simulink library "libsb2sl"  (Simulink 7.3)
settings: Solver=ode45  SolverMode=SingleTasking  StartTime=0.0  StopTime=10.0  RelTol=1e-3
PostLoadFcn:
  | setsysloc libsb2sl
undefined symbols (not defined in the file): A, Ac, Ad, B, Bc, Bd, C, Cc, Cd, code, const, D, data, Dc, Dd, DiscIntNeverNeededParam, gain, info, k, m, map, no, stat, X0, xd, xi
libraries: simulink3 x17, simulink x5, libsb2sl x3
(part 1 of 3)
Description:
  | Translation blocks
  | 
  | Copyright 1997-2008 The MathWorks, Inc.
settings Model: Creator=alex  LastModifiedBy=sgage  ExtModeAutoUpdateStatusClock=off
settings Model: ForwardingTableString=|
  | ||__slOldName__||libsb2sl/TRN/Sph2Cart||__slNewName__||simulink_extras/Transformations/Spherical to
  | Cartesian||__slOldName__||libsb2sl/TRN/Cart2Sph||__slNewName__||simulink_extras/Transformations/Cartesian to
  | Spherical||__slOldName__||libsb2sl/TRN/Polar2Cart||__slNewName__||simulink_extras/Transformations/Polar to
  | Cartesian||__slOldName__||libsb2sl/TRN/Cart2Polar||__slNewName__||simulink_extras/Transformations/Cartesian to
  | Polar||__slOldName__||libsb2sl/ALG/DotProduct||__slNewName__||simulink/Math
  | Operations/Dot Product

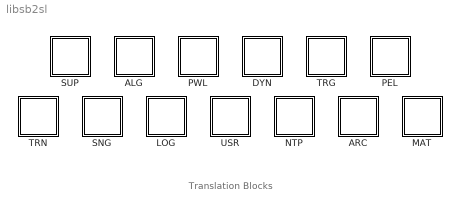
== system libsb2sl ==
  note: Translation Blocks
  ALG : Subsystem
  ARC : Subsystem
  DYN : Subsystem
  LOG : Subsystem
  MAT : Subsystem  AncestorBlock=libsb2sl/ARC
  NTP : Subsystem
  PEL : Subsystem
  PWL : Subsystem
  SNG : Subsystem
  SUP : Subsystem
  TRG : Subsystem
  TRN : Subsystem
  USR : Subsystem

== system libsb2sl/ALG ==
  1VarPoly : S-Function  FunctionName=sb1varpoly  Parameters=COEFF  EnableBusSupport=off  mask(ALG-Palette){COEFF=[1 2]}
      mask prompts: COEFF "Coefficients:"
      mask init:
      | [x,y]=sblibico('polyOneVar');
      mask Display: plot(0,0,1,1,x,y)
  AlgExpression : Subsystem
  CrossProd : Subsystem  mask(ALG-Palette){}
      mask help: Cross-product multiplication.
      mask init:
      | [x,y]=sblibico('crossProduct');
      mask Display: plot(0,0,1,1,x,y)

== system libsb2sl/ARC ==
  BreakPoints : Subsystem  mask(ARC-Palette){BrkPoints=[-1 1;0 2;1 3]}
      mask prompts: BrkPoints "Breakpoint Matrix:"
      mask help: Linear Interpolation.
      mask init:
      | % LinInterp MaskInit code
      | [x,y]=sblibico('linearInterp');
      | in1BrkPoints=BrkPoints(:,1:2:end);
      | outBrkPoints=BrkPoints(:,2:2:end);
      mask Display: plot(0,0,1,1,x,y)
  InterpTable : Subsystem  mask(ARC-Palette){numInp=One, BrkPoints=[-5:5; -5:5; -10:2:10]'}
      mask prompts: numInp "Number of Inputs:"; BrkPoints "Interpolation Table:"
      mask help: Linear Interpolation Table.
      mask init:
      | if (numInp==1)
      | in1BrkPoints=BrkPoints(:,1);
      | in2BrkPoints=[1:size(BrkPoints,2)-1];
      | outBrkPoints=BrkPoints(:,2:end);
      | [x,y]=sblibico('linearInterp');
      | else
      | in1BrkPoints=BrkPoints(1:end-1,1);
      | in2BrkPoints=BrkPoints(end,2:end);
      | outBrkPoints=BrkPoints(1:end-1,2:end);
      | [x,y]=sblibico('bilinearInterp');
      | end
      mask StyleString: popup(One|Two),edit
      mask Display: plot(0,0,1,1,x,y)

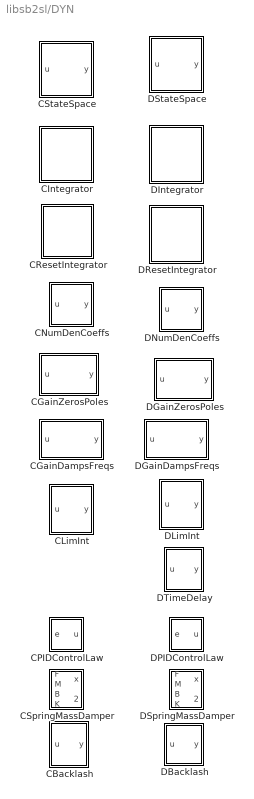
== system libsb2sl/DYN ==
  CBacklash : Subsystem  mask(DYN-Palette){W=1, N=1, X0=0, Wc=1}
      mask prompts: W "Backlash Width:"; N "Backlash Slope:"; X0 "Initial Conditions:"; Wc "Cutoff Frequency:"
      mask help: A non-linear dynamic system that models hysteresis.
      mask init:
      | lb=-0.5*W; ub=-lb;
      | [x,y]=sblibico('backlash');
      mask Display: plot(0,0,1,1,x,y)
  CGainDampsFreqs : Subsystem  mask(DYN-Palette){G=1, Xz=[], Wz=[], Xp=[0.7], Wp=[1], Y0=0}
      mask prompts: G "Gain:"; Xz "Zeros-Damping Ratios:"; Wz "Zeros-Natural Frequencies:"; Xp "Poles-Damping Ratios:"; Wp "Poles-Natural Frequencies:"; Y0 "Initial Output:"
      mask help: Transfer function in damping ratios and natural frequencies.
      mask init:
      | [A,B,C,D]=sblibdrv('CmplxZP',G,Xz,Wz,Xp,Wp,0);
      | if (isempty(Y0)), Y0 = zeros(1,size(C,1)); end;
      | X0=C\Y0;
      | [x,y]=sblibico('gainDampsFreq','cont');
      mask Display: plot(0,0,1,1,x,y)
  CGainZerosPoles : Subsystem  mask(DYN-Palette){K=1, Z=1, P=-1, Y0=0}
      mask prompts: K "Gain:"; Z "Zeros:"; P "Poles:"; Y0 "Initial Output:"
      mask help: Transfer function expressed in real poles and real zeros.
      mask init:
      | [A,B,C,D]=zp2ss(Z,P,K);
      | if (isempty(Y0)), X0 = zeros(1,size(C,1)); end;
      | X0=C\Y0;
      | [x,y]=sblibico('gainZerosPoles','cont');
      mask Display: plot(0,0,1,1,x,y)
  CIntegrator : Subsystem
  CLimInt : Subsystem  mask(DYN-Palette){UB=5, LB=-5, K=1, X0=5}
      mask prompts: UB "Upper Limit:"; LB "Lower Limit:"; K "Gain:"; X0 "Initial condition:"
      mask init:
      | [x,y]=sblibico('limIntegrator','cont');
      mask Display: plot(0,0,1,1,x,y)
  CNumDenCoeffs : Subsystem  mask(DYN-Palette){NU=2, NUM=[1 2;1.1 1], DEN=[0.5  1], Y0=[0.5;0.5]}
      mask prompts: NU "Number of Inputs:"; NUM "Numerator:"; DEN "Denominator:"; Y0 "Initial Output:"
      mask help: Transfer function in numerator-denominator form.
      mask init:
      | if (isempty(NU)), NU=1; end
      | [Ac,Bc,Cc,Dc] = sblibdrv('NumDen',NUM,DEN,NU);
      | if (isempty(Y0)); Y0=zeros(1,size(Cc,1)); end
      | X0=Cc\Y0(:);
      | [x,y]=sblibico('numDenCoeffs','cont');
      mask Display: plot(0,0,1,1,x,y)
  CPIDControlLaw : Subsystem  mask(DYN-Palette){P=1, I=1, D=0, TAU=0, X0=0}
      mask prompts: P "Proportional Gain:"; I "Integral Gain:"; D "Derivative Gain:"; TAU "Derivative Time Constant:"; X0 "Initial Conditions:"
      mask help: PID Control Law.
      mask init:
      | if (exist('X0')==0),X0=[];end
      | [xi,xd]=sblibdrv('pidControl',I,D,TAU,X0);
      | [x,y]=sblibico('pidControl');
      mask Display: plot(0,0,1,1,x,y)
  CResetIntegrator : Subsystem
  CSpringMassDamper : Subsystem  mask(DYN-Palette){X0=[0,0]}
      mask prompts: X0 "Initial Conditions:"
      mask help: Spring Mass Damper.
      mask init:
      | [x,y]=sblibico('springMassDamper');
      mask Display: plot(0,0,1,1,x,y)
  CStateSpace : Subsystem  mask(DYN-Palette){NX=1, SYS=[1 1;1 0], X0=[]}
      mask prompts: NX "Number of States:"; SYS "System Matrix:"; X0 "Initial Conditions:"
      mask help: State-space system.
      mask init:
      | if (~exist('X0','var')), X0=[]; end
      | if isempty(X0), X0=zeros(NX,1); end
      | NX1=NX+1;
      | A=SYS(1:NX,1:NX);
      | B=SYS(1:NX,NX1:end);
      | C=SYS(NX1:end,1:NX);
      | D=SYS(NX1:end,NX1:end);
      | [x,y]=sblibico('stateSpace','cont');
      mask Display: plot(0,0,1,1,x,y)
  DBacklash : Subsystem  mask(DYN-Palette){W=1, N=1, X0=0, TS=1}
      mask prompts: W "Backlash Width:"; N "Backlash Slope:"; X0 "Initial Conditions:"; TS "Sampling Time:"
      mask help: A non-linear dynamic system that models hysteresis.
      mask init:
      | lb=-0.5*W; ub=-lb;
      | [x,y]=sblibico('backlash');
      mask Display: plot(0,0,1,1,x,y)
  DGainDampsFreqs : Subsystem  mask(DYN-Palette){G=1, Xz=[], Wz=[], Xp=0.7, Wp=1, Y0=0, TS=0.1}
      mask prompts: G "Gain:"; Xz "Zeros-Damping Ratios:"; Wz "Zeros-Natural Frequencies:"; Xp "Poles-Damping Ratios:"; Wp "Poles-Natural Frequencies:"; Y0 "Initial Output:"; TS "Sample Time:"
      mask help: Transfer function in damping ratios and natural frequencies.
      mask init:
      | [A,B,C,D]=sblibdrv('CmplxZP',G,Xz,Wz,Xp,Wp,TS(1));
      | if (isempty(Y0)), Y0 = zeros(1,size(C,1)); end;
      | X0=C\Y0;
      | [x,y]=sblibico('gainDampsFreq','disc');
      mask Display: plot(0,0,1,1,x,y)
  DGainZerosPoles : Subsystem  mask(DYN-Palette){K=1, Z=[], P=-1, Y0=0, TS=1}
      mask prompts: K "Gain:"; Z "Zeros:"; P "Poles:"; Y0 "Initial Output:"; TS "Sample Time:"
      mask help: Transfer function expressed in real poles and real zeros.
      mask init:
      | [A,B,C,D]=zp2ss(Z,P,K);
      | if (isempty(Y0)), Y0 = zeros(1,size(C,1)); end;
      | X0=C\Y0;
      | [x,y]=sblibico('gainZerosPoles','disc');
      mask Display: plot(0,0,1,1,x,y)
  DIntegrator : Subsystem
  DLimInt : Subsystem  mask(DYN-Palette){IMODE=ForwardEuler, UB=5, LB=-5, K=1, X0=0, TS=0.1}
      mask prompts: IMODE "Integrator Method:"; UB "Upper Limit:"; LB "Lower Limit:"; K "Gain:"; X0 "Initial Conditions:"; TS "Sampling Period:"
      mask init:
      | method={'ForwardEuler';'BackwardEuler';'Trapezoidal'};
      | set_param([gcb '/Integrator'],'IntegratorMethod',method{IMODE});
      | [x,y]=sblibico('limIntegrator','disc');
      mask StyleString: popup(ForwardEuler|BackwardEuler|Trapezoidal),edit,edit,edit,edit,edit
      mask Display: plot(0,0,1,1,x,y)
  DNumDenCoeffs : Subsystem  mask(DYN-Palette){NU=2, NUM=[1 2;1.1 1], DEN=[0.5  1], Y0=-[0.5;0.5], TS=0.1}
      mask prompts: NU "Number of Inputs:"; NUM "Numerator:"; DEN "Denominator:"; Y0 "Initial Output:"; TS "Sample Time:"
      mask help: Transfer function in numerator-denominator form.
      mask init:
      | if (isempty(NU)), NU=1; end
      | [Ad,Bd,Cd,Dd]=sblibdrv('NumDen',NUM,DEN,NU);
      | if (isempty(Y0)); Y0=zeros(1,size(Cd,1)); end
      | X0=Cd\Y0(:);
      | [x,y]=sblibico('numDenCoeffs','disc');
      mask Display: plot(0,0,1,1,x,y)
  DPIDControlLaw : Subsystem  mask(DYN-Palette){P=1, I=1, D=0, TAU=0, X0=0, TS=1}
      mask prompts: P "Proportional Gain:"; I "Integral Gain:"; D "Derivative Gain:"; TAU "Derivative Time Constant:"; X0 "Initial Conditions:"; TS "Sampling Period:"
      mask help: PID Control Law.
      mask init:
      | if (exist('X0')==0),X0=[];end
      | [xi,xd]=sblibdrv('pidControl',I,D,TAU,X0);
      | [x,y]=sblibico('pidControl');
      mask Display: plot(0,0,1,1,x,y)
  DResetIntegrator : Subsystem
  DSpringMassDamper : Subsystem  mask(DYN-Palette){X0=[0,0], TS=0.01}
      mask prompts: X0 "Initial Conditions:"; TS "Sampling Period:"
      mask help: Spring Mass Damper.
      mask init:
      | if (length(TS)==1),TS(2)=0;end
      | [x,y]=sblibico('springMassDamper');
      mask Display: plot(0,0,1,1,x,y)
  DStateSpace : Subsystem  mask(DYN-Palette){NX=1, SYS=[1 1;1 0], X0=[], TS=1}
      mask prompts: NX "Number of States:"; SYS "System Matrix:"; X0 "Initial Conditions:"; TS "Sampling Time:"
      mask init:
      | if (~exist('X0','var')), X0=[]; end
      | if isempty(X0), X0=zeros(NX,1); end
      | NX1=NX+1;
      | A=SYS(1:NX,1:NX);
      | B=SYS(1:NX,NX1:end);
      | C=SYS(NX1:end,1:NX);
      | D=SYS(NX1:end,NX1:end);
      | [x,y]=sblibico('stateSpace','disc');
      mask Display: plot(0,0,1,1,x,y)
  DTimeDelay : Subsystem  mask(DYN-Palette){TAU=1.1, Y0=0, TS=1}
      mask prompts: TAU "Time Delay:"; Y0 "Initial Output:"; TS "Sampling Time:"
      mask init:
      | if (isempty(Y0)), Y0=0; end;
      | [k,m,no,X0]=sblibdrv('dDelay',TAU,Y0,TS);
      | [x,y]=sblibico('timeDelay');
      mask Display: plot(0,0,1,1,x,y)

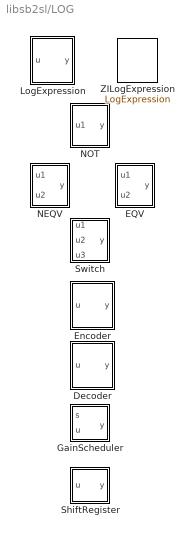
== system libsb2sl/LOG ==
  Decoder : Subsystem  mask(LOG-Palette){BPI=4, MIN=-1, MAX=1}
      mask prompts: BPI "Number of Bits per Input:"; MIN "Input Minimum:"; MAX "Input Maximum:"
      mask help: Decimal to binary conversion.
      mask init:
      | [x,y]=sblibico('decoder');
      mask Display: plot(0,0,1,1,x,y)
  EQV : Subsystem  mask(LOG-Palette){}
      mask help: Logical operator EQV.
      mask init:
      | [x,y]=sblibico('logOperator','EQV');
      mask Display: plot(0,0,1,1,x,y)
  Encoder : Subsystem  mask(LOG-Palette){BPO=4, MIN=-1, MAX=1}
      mask prompts: BPO "Number of Bits per Output:"; MIN "Output Minimum:"; MAX "Output Maximum:"
      mask help: Binary to decimal conversion.
      mask init:
      | [x,y]=sblibico('encoder');
      mask Display: plot(0,0,1,1,x,y)
  GainScheduler : Subsystem  mask(LOG-Palette){IND=[-1,0,1], GAIN=[1,2,3]}
      mask prompts: IND "Switch Breakpoints:"; GAIN "Gain Matrices:"
      mask help: Gain scheduler
      mask init:
      | [x,y]=sblibico('gainSched');
      mask Display: plot(0,0,1,1,x,y)
  LogExpression : Subsystem  mask(LOG-Palette){SRC='y1=u1;y2=t;', P0=[], TS=-1}
      mask prompts: SRC "Logical and Relational Equations:"; P0 "Initial Parameter Values:"; TS "Sampling Period:"
      mask help: Logical expressions.
      mask init:
      | if (exist('P0')==0),P0=[];end
      | [src,stat,code,data,info]=sblibdrv('LogicalExp',SRC,P0);
      mask Display: text(0.1,0.5,src,'HorizontalAlignment','left')
  NEQV : Subsystem  mask(LOG-Palette){}
      mask help: Logical operator NEQV.
      mask init:
      | [x,y]=sblibico('logOperator','NEQV');
      mask Display: plot(0,0,1,1,x,y)
  NOT : Subsystem  mask(LOG-Palette){}
      mask help: Logical operator NOT.
      mask init:
      | [x,y]=sblibico('logOperator','NOT');
      mask Display: plot(0,0,1,1,x,y)
  ShiftRegister : Subsystem  mask(LOG-Palette){NX=1, NY=1, X0=0, TS=1}
      mask prompts: NX "Number of Stages:"; NY "Number of  Output Stages:"; X0 "Initial Values:"; TS "Sampling Time:"
      mask help: Sequential Shift Register
      mask init:
      | if (~exist('X0','var')), X0=[]; end
      | if (isempty(X0)), X0=zeros(NX,1); end
      | [x,y]=sblibico('shiftReg');
      mask Display: plot(0,0,1,1,x,y)
  Switch : Subsystem
      mask Type: LOG-Palette
      mask Description: Switches between two data sources.
      mask Display: plot(0,1.2,10,10.5,[0 5 5 4.5 5.5 5],[9 9 4 5.5 5.5 4],[0 3],[6 6],[0 3 8 10],[3 3 6 6])
  ZILogExpression : libsb2sl/LOG/LogExpression  SystemSampleTime=-1  SRC='y1=u1;y2=t;'  P0=[]  TS=-1

== system libsb2sl/MAT ==
  Constant : Subsystem  mask(MAT-Palette){constantName='H', constantValue=[1,1;2,4];}
      mask prompts: constantName "Constant Name:"; constantValue "Constant Value:"
      mask init:
      | if (~exist('constantName','var')), constantName='';end
      | if (isempty(constantName)), constantName='H';end
      | if (~ischar(constantName)), constantName=char(constantName);end
      | if (any(size(constantValue) > 1)), constantValue=constantValue.';constantValue=constantValue(:);end
      mask Display: disp(constantName)
  LeftMultiply : Subsystem  mask(MAT-Palette){G=[5 10], dimMatrixA=[2,2]}
      mask prompts: G "Gain:"; dimMatrixA "Matrix A Dimension:"
      mask init:
      | [x,y]=sblibico('matLeftMul');
      | nARows=dimMatrixA(1);nACols=dimMatrixA(2);
      | [nGRows,nGCols]=size(G);
      | G=G.';
      | if (nGCols ~= nARows)
      | error('Inner matrix dimensions must agree.');
      | end
      mask Display: plot(0,0,1,1,x,y)
  MatLeftDivide : Subsystem  mask(MAT-Palette){dimMatrixA=[2,2], dimMatrixB=[2,2]}
      mask prompts: dimMatrixA "Matrix A Dimension:"; dimMatrixB "Matrix B Dimension:"
      mask init:
      | [x,y]=sblibico('matLeftDiv');
      | nARows=dimMatrixA(1);nACols=dimMatrixA(2);
      | nBRows=dimMatrixB(1);nBCols=dimMatrixB(2);
      | if (nACols ~= nBRows)
      | error('Matrix dimensions must agree.');
      | end
      mask Display: plot(0,0,1,1,x,y)
  MatRightDivide : Subsystem  mask(MAT-Palette){dimMatrixA=[2,2], dimMatrixB=[2,2]}
      mask prompts: dimMatrixA "Matrix A Dimension:"; dimMatrixB "Matrix B Dimension:"
      mask init:
      | [x,y]=sblibico('matRightDiv');
      | nARows=dimMatrixA(1);nACols=dimMatrixA(2);
      | nBRows=dimMatrixB(1);nBCols=dimMatrixB(2);
      | if (nARows ~= nBCols)
      | error('Matrix dimensions must agree.');
      | end
      mask Display: plot(0,0,1,1,x,y)
  MatrixInverse : Subsystem  mask(MAT-Palette){dimMatrixA=[2,2]}
      mask prompts: dimMatrixA "Matrix A Dimension:"
      mask init:
      | [x,y]=sblibico('matInverse');
      | nARows=dimMatrixA(1);nACols=dimMatrixA(2);
      mask Display: plot(0,0,1,1,x,y)
  MatrixMultiply : Subsystem  mask(MAT-Palette){dimMatrixA=[2,2], dimMatrixB=[2,2]}
      mask prompts: dimMatrixA "Matrix A Dimension:"; dimMatrixB "Matrix B Dimension:"
      mask init:
      | [x,y]=sblibico('matMultiply');
      | nARows=dimMatrixA(1);nACols=dimMatrixA(2);
      | nBRows=dimMatrixB(1);nBCols=dimMatrixB(2);
      | if (nACols ~= nBRows)
      | error('Inner matrix dimensions must agree.');
      | end
      mask Display: plot(0,0,1,1,x,y)
  MatrixTranspose : Subsystem  mask(MAT-Palette){dimMatrixA=[2,2]}
      mask prompts: dimMatrixA "Matrix A Dimension:"
      mask init:
      | [x,y]=sblibico('matTrans');
      | nARows=dimMatrixA(1);nACols=dimMatrixA(2);
      | if ((nARows==1)|(nACols==1)),
      | mapIndices=1:nARows*nACols;
      | else
      | mapMatrix=[1:nACols;nACols*ones(nARows-1,nACols)];
      | mapIndices=cumsum(mapMatrix);
      | end
      mask Display: plot(0,0,1,1,x,y)
  RightMultiply : Subsystem  mask(MAT-Palette){dimMatrixA=[2,2], G=[5; 10]}
      mask prompts: dimMatrixA "Matrix A Dimension:"; G "Gain:"
      mask init:
      | [x,y]=sblibico('matRightMul');
      | nARows=dimMatrixA(1);nACols=dimMatrixA(2);
      | [nGRows,nGCols]=size(G);
      | G=G.';
      | if (nACols ~= nGRows)
      | error('Inner matrix dimensions must agree.');
      | end
      mask Display: plot(0,0,1,1,x,y)

== system libsb2sl/NTP ==
  BiCubicInterp : Subsystem  mask(NTP-Palette){in1BrkPoints=[-1,1], in2BrkPoints=[-1,0,1], outBrkPoints=[-1,1;-1,1;-1,1]}
      mask prompts: in1BrkPoints "Input-1 Breakpoints:"; in2BrkPoints "Input-2 Breakpoints:"; outBrkPoints "Output Values:"
      mask help: Bicubic interpolation.
      mask init:
      | % BiCubicInterp MaskInit code
      | [x,y]=sblibico('bicubicInterp');
      mask Display: plot(0,0,1,1,x,y)
  BiLinearInterp : Subsystem  mask(NTP-Palette){in1BrkPoints=[-1,1], in2BrkPoints=[-1,0,1], outBrkPoints=[-1,1;-1,1;-1,1]}
      mask prompts: in1BrkPoints "Input-1 Breakpoints:"; in2BrkPoints "Input-2 Breakpoints:"; outBrkPoints "Output Values:"
      mask help: Bilinear interpolation.
      mask init:
      | % BiLinInterp MaskInit code
      | [x,y]=sblibico('bilinearInterp');
      | 
      | % Set up for sfun_lookupnd input
      | bpData = [in2BrkPoints(:); in1BrkPoints(:)];  % Note: row major!
      | bpIndices_uint32 = uint32([0, length(in2BrkPoints)]);
      | searchMode = 2;
      | cacheBpFlag = 1;
      | tableData = outBrkPoints;
      | numDims = 2;
      | interpMethod = 2;
      | extrapMethod = 2;
      | rangeErrorMode = 1;
      | vectorInputFlag = 0;
      mask Display: plot(0,0,1,1,x,y)
  ConstantInterp : Subsystem  mask(NTP-Palette){in1BrkPoints=[-1,0,1], outBrkPoints=[1,2,3]}
      mask prompts: in1BrkPoints "Input Breakpoints:"; outBrkPoints "Output Values:"
      mask help: Constant Interpolation.
      mask init:
      | % ConstantInterp MaskInit code
      | [x,y]=sblibico('constInterp');
      mask Display: plot(0,0,1,1,x,y)
  CubicInterp : Subsystem  mask(TRN-Palette){in1BrkPoints=[-1,0,1], outBrkPoints=[1,2,3]}
      mask prompts: in1BrkPoints "Input Breakpoints:"; outBrkPoints "Output Values:"
      mask help: Cubic Spline Interpolation
      mask init:
      | %CubicInterp MaskInit code
      | [x,y]=sblibico('cubicInterp');
      mask Display: plot(0,0,1,1,x,y)
  LinearInterp : Subsystem  mask(TRN-Palette){in1BrkPoints=[-1,0,1], outBrkPoints=[1,2,3]}
      mask prompts: in1BrkPoints "Input Breakpoints:"; outBrkPoints "Output Values:"
      mask help: Linear Interpolation.
      mask init:
      | % LinInterp MaskInit code
      | [x,y]=sblibico('linearInterp');
      mask Display: plot(0,0,1,1,x,y)
  MultiLinearInterp : Subsystem  mask(NTP-Palette){NINP=2, in1BrkPoints=[1,2], in2BrkPoints=[1,2], in3BrkPoints=3, in4BrkPoints=4, in5BrkPoints=5, in6BrkPoints=6, in7BrkPoints=7, in8BrkPoints=8, outBrkPoints=[1,2;3,4]}
      mask prompts: NINP "Number of  Inputs:"; in1BrkPoints "Input-1 Breakpoints:"; in2BrkPoints "Input-2 Breakpoints:"; in3BrkPoints "Input-3 Breakpoints:"; in4BrkPoints "Input-4 Breakpoints:"; in5BrkPoints "Input-5 Breakpoints:"; in6BrkPoints "Input-6 Breakpoints:"; in7BrkPoints "Input-7 Breakpoints:"; in8BrkPoints "Input-8 Breakpoints:"; outBrkPoints "Output Values:"
      mask help: Multilinear interpolation.
      mask init:
      | % MultiLinInterp MaskInit code
      | [x,y]=sblibico('mdlinearInterp',NINP);
      | 
      | % Set up for sfun_lookupnd input
      | bpSizes = zeros(1,NINP+1);
      | bpSizes(1) = length(in1BrkPoints);
      | for i = 1:NINP,  % NINP is 1 for 2D, 2 for 3D, etc.
      |   bpDataNext = eval(['in' num2str(i+1) 'BrkPoints(:)']);
      |   bpSizes(i+1) = length(bpDataNext);
      |  end
      | tableData = reshape(outBrkPoints,bpSizes);
      mask StyleString: popup(2|3|4|5|6|7|8),edit,edit,edit,edit,edit,edit,edit,edit,edit
      mask CallbackString: sblibdrv('MultiLin','mask',gcb);|||||||||
      mask Display: plot(0,0,1,1,x,y)

== system libsb2sl/PEL ==
  Constant**u : Subsystem  mask(PEL-Palette){CONST=5}
      mask prompts: CONST "Constant:"
      mask init:
      | [x,y]=sblibico('constantU');
      mask Display: plot(0,0,1,1,x,y)
  SignedSqrt : Subsystem  mask(PEL-Palette){}
      mask init:
      | [x,y]=sblibico('signedSqrt');
      mask Display: plot(0,0,1,1,x,y)
  u**Constant : Subsystem  mask(PEL-Palette){CONST=5}
      mask prompts: CONST "Constant:"
      mask init:
      | [x,y]=sblibico('uConstant');
      mask Display: plot(0,0,1,1,x,y)

== system libsb2sl/PWL ==
  Preload : Subsystem  mask(PWL-Palette){preload=[1 3 2 0], slope=1}
      mask help: Performs preload or Coulomb switch function.
      mask init:
      | x=max(preload(1),slope(1)+preload(1));
      mask Display: plot([-1 0 0 1],[-slope(1)-preload(1),-preload(1),preload(1), slope(1)+preload(1)],[-1 1],[0 0],[0 0],[-x,x])
  Quantization : Subsystem  mask(PWL-Palette){RES=1, OPER=round}
      mask prompts: RES "Resolution:"; OPER "Type"
      mask init:
      | x=[-3:0.1:3];operator={'round';'fix';'floor';'ceil'};
      | y=feval(operator{OPER},x);
      | [xx,yy]=stairs(x,y);
      | set_param([gcb '/Type'],'Operator',operator{OPER});
      mask StyleString: edit,popup(round|truncate|floor|ceil)
      mask Display: plot([0 0],[-3,3],[-3,3],[0 0],xx,yy)

== system libsb2sl/SNG ==
  CNormalRandom : Subsystem  mask(SGN-Palette){SEED=0, T0=0, MEAN=0, STD=1, INTM=Linear, TS=1}
      mask prompts: T0 "Relative Start Time:"; STD "Standard Deviation:"; INTM "Interpolation Method:"; TS "Output Interval:"
      mask help: Random Number Generator, Normal
      mask init:
      | start=sscanf(get_param(bdroot(gcs),'StartTime'),'%g')+T0;
      mask StyleString: edit,edit,edit,edit,popup(Constant|Linear),edit
      mask Display: plot([-1,11],[0,0],[0,0],[-0.1,1],[0:10],rand(1,11))
  CUniformRandom : Subsystem  mask(SGN-Palette){SEED=1, T0=0, MIN=0, MAX=1, INTM=Constant, TS=1}
      mask prompts: T0 "Relative Start Time:"; MIN "Minimum:"; MAX "Maximum:"; INTM "Interpolation Method:"; TS "Output Interval:"
      mask help: Random Number Generator, Uniform.
      mask init:
      | start=sscanf(get_param(bdroot(gcs),'StartTime'),'%g')+T0;
      mask StyleString: edit,edit,edit,edit,popup(Constant|Linear),edit
      mask Display: plot([-1,11],[0,0],[0,0],[-0.1,1],[0:10],rand(1,11))
  DNormalRandom : Subsystem  mask(SGN-Palette){SEED=0, T0=0, MEAN=0, STD=1, TS=1}
      mask prompts: T0 "Relative Start Time:"; STD "Standard Deviation:"; TS "Sampling Time:"
      mask help: Random Number Generator, Normal
      mask init:
      | start=sscanf(get_param(bdroot(gcs),'StartTime'),'%g')+T0;
      mask Display: plot([-1,11],[0,0],[0,0],[-0.1,1],[0:10],rand(1,11))
  DUniformRandom : Subsystem  mask(SGN-Palette){SEED=1, T0=0, MIN=0, MAX=1, TS=1}
      mask prompts: T0 "Relative Start Time:"; MIN "Minimum:"; MAX "Maximum:"; TS "Sampling Time:"
      mask help: Random Number Generator, Uniform.
      mask init:
      | start=sscanf(get_param(bdroot(gcs),'StartTime'),'%g')+T0;
      mask Display: plot([-1,11],[0,0],[0,0],[-0.1,1],[0:10],rand(1,11))
  GenWaveform : Subsystem  mask(SGN-Palette){T0=0.6, TAC=[0 1 2], SAC=[0 0;1 2;0 0]}
      mask prompts: T0 "Relative Start Time:"; TAC "Time Values:"; SAC "Output Values:"
      mask help: General Waveform.
      mask init:
      | in1BrkPoints=TAC(:);
      | outBrkPoints=SAC;
      | period = max(in1BrkPoints);
      | start=sscanf(get_param(bdroot(gcs),'StartTime'),'%g')+T0;
      mask Display: plot([1,1,1,11],[-1,2,0,0],[3,4,4.5,5,6,7,8,8.5,9,10,11],[0,1,0.8,1.5,-0.5,0,1,0.8,1.5,-0.5,0])
  LimRamp : Subsystem  mask(SGN-Palette){T0=[2 4], RATE=[1 -1], LMT=no, SAT=[]}
      mask prompts: T0 "Relative Start Time:"; RATE "Ramp Signal Slope:"; LMT "Should Ramp be Limited?"; SAT "Ramp Saturation:"
      mask help: Ramp (Limited)
      mask init:
      | if (LMT==1),SAT=RATE*(sscanf(get_param(bdroot(gcs),'StopTime'),'%g')+1);end;
      | start=sscanf(get_param(bdroot(gcs),'StartTime'),'%g')+T0;
      mask StyleString: edit,edit,popup(no|yes),edit
      mask Display: plot([1,1,1,10],[-1,6,0,0],[3,9,10],[0,5,5])
  PulseTrain : Subsystem  mask(SNG-Palette){T0=[2 3], A=[1 0.8], PW=[0.2 0.1], F=[0.5 0.8]}
      mask prompts: T0 "Relative Start Time:"; A "Pulse Magnitude:"; PW "Pulse Width in sec:"; F "Pulse Frequency in Hz:"
      mask help: Pulse Train.
      mask init:
      | start=T0+sscanf(get_param(bdroot(gcs),'StartTime'),'%g');
      mask Display: plot([1,1,1,12],[-1,2,0,0],[3,3,4,4,6,6,7,7,9,9,10,10,12],[0,1,1,0,0,1,1,0,0,1,1,0,0])
  SinusoidGen : Subsystem  mask(SGN-Palette){T0=[2 4], A=[1 1.6], PHI=[0 90], F=[1 2]}
      mask prompts: T0 "Relative Start Time:"; A "Signal Magnitude:"; PHI "Phase Angle in Degrees:"; F "Sinusoid Frequency in Hz:"
      mask help: Sinusoid Generator.
      mask init:
      | start=sscanf(get_param(bdroot(gcs),'StartTime'),'%g')+T0;
      mask Display: plot([1,1,1,10],[-2,2,0,0],3:0.1:10,1.5*sin(0:0.1:7))
  SquareWave : Subsystem  mask(SGN-Palette){T0=[0.6 0.8], A=[1.9 1], PW=[0.5 0.85], PF=[1 0.25]}
      mask prompts: T0 "Relative Start Time:"; A "Pulse Magnitude:"; PW "Pulse Width:"; PF "Pulse Frequency:"
      mask help: Square Wave.
      mask init:
      | ind=find(PF==0);if isempty(ind),period=1.0./PF;else PF(ind)=1;period=1.0./PF;period(ind)=sscanf(get_param(bdroot(gcs),'StopTime'),'%g')+1;end
      | in1BrkPoints=[zeros(size(PW));PW];
      | outBrkPoints=[A;-A];
      | start=sscanf(get_param(bdroot(gcs),'StartTime'),'%g')+T0;
      mask Display: plot([1,1,1,10],[-2,2,0,0],[3,3,5,5,6,6,8,8,9,9,10],[0,1,1,-1,-1,1,1,-1,-1,1,1])
  StepFcn : Subsystem  mask(SGN-Palette){T0=2, A=1, TS=0}
      mask prompts: T0 "Relative Start Time:"; A "Step Magnitude:"; TS "Sampling Time:"
      mask help: Step Function
      mask init:
      | start=sscanf(get_param(bdroot(gcs),'StartTime'),'%g')+T0;
      mask Display: plot([1,1,1,8],[-1,2,0,0],[3,3,8],[0,1,1])

== system libsb2sl/SUP ==
  ConditionBlock : S-Function  FunctionName=sbcondlog  Parameters=MODE  EnableBusSupport=off  mask(SUP-Palette){MODE=No Default}
      mask help: Condition Block.
      mask init:
      | [x,y]=sblibico('condBlock');
      mask StyleString: popup(No Default|With Default|Sequential)
      mask Display: plot(0,0,1,1,x,y)
  DataStoreRW : Subsystem  mask(SUP-Palette){MLOC=VAR, NREG=4, RIND=[], TS=1}
      mask prompts: MLOC "Data Store Name:"; NREG "Number of Registers:"; RIND "Input Indices:"; TS "Sampling Time:"
      mask help: Data store.
      mask init:
      | [x,y]=sblibico('dataStore');
      | if (~exist('RIND','var')), RIND=[]; end
      | [inpWidth,inputMap]=sblibdrv('DataStore',NREG,RIND);
      | set_param([gcb '/dsRead'],'DataStoreName',MLOC);
      | set_param([gcb '/dsWrite'],'DataStoreName',MLOC);
      mask Display: plot(0,0,1,1,x,y)
  DataStoreW : Subsystem  mask(SUP-Palette){MLOC=VAR, NREG=4, RIND=[], TS=1}
      mask prompts: MLOC "Data Store Name:"; NREG "Number of Registers:"; RIND "Input Indices:"; TS "Sampling Time:"
      mask help: Data store.
      mask init: same as libsb2sl/SUP/DataStoreRW
      mask Display: plot(0,0,1,1,x,y)

== system libsb2sl/TRG ==
  CosAsin : Subsystem
      mask Type: TRG-Palette
      mask Description: Cosine of the arcsine of the input.
      mask Display: disp('cos(asin)')
  CosAtan2 : Subsystem
      mask Type: TRG-Palette
      mask Description: Cosine of arctangent of two inputs.
      mask Display: disp('cos(atan2)')
  SinAtan2 : Subsystem
      mask Type: TRG-Palette
      mask Description: Sine of arctangent of two inputs.
      mask Display: disp('sin(atan2)')

== system libsb2sl/TRN ==
  DAxisRotation : S-Function  FunctionName=sbdaxisrot  Parameters=SEQ  EnableBusSupport=off  mask(TRN-Palette){SEQ=[1 2 3]}
      mask prompts: SEQ "Axis Sequence:"
      mask init:
      | if isempty(SEQ), SEQ=[1 2 3]; end
      | [x,y]=sblibico('dirAxisRot');
      mask Display: plot(0,0,1,1,x,y)
  IAxisRotation : S-Function  FunctionName=sbiaxisrot  Parameters=SEQ  EnableBusSupport=off  mask(TRN-Palette){SEQ=[1 2 3]}
      mask prompts: SEQ "Axis Sequence:"
      mask init:
      | if isempty(SEQ), SEQ=[1 2 3]; end
      | [x,y]=sblibico('invAxisRot');
      mask Display: plot(0,0,1,1,x,y)

== system libsb2sl/USR ==
  BlockScript : Subsystem  mask(USR-Palette){BSNAME=foo, SIZES=[1 1 1], BSPARA=, BSARGS=, X0=0}
      mask prompts: BSNAME "Blockscript Name:"; BSPARA "Parameter Names:"; BSARGS "Blockscript Parameters:"; X0 "Initial Conditions:"
      mask help: BlockScript Programming Language.
      mask init:
      | if isempty(X0), X0=0;end
      | if isempty(BSPARA),
      | set_param([gcb '/BlockScriptCode'],'FunctionName',BSNAME,'Parameters',cat(2,'SIZES,X0'));
      | else ARGS=evalin('base',cat(2,'{',BSARGS,'}'));
      | eval(cat(2,'[',BSPARA,']=deal(ARGS{:});'));
      | set_param([gcb '/BlockScriptCode'],'FunctionName',BSNAME,'Parameters',cat(2,'SIZES,',BSPARA,',X0')); end
      mask Display: fprintf('Block\nScript')
  ZIBlockScript : Subsystem  mask(USR-Palette){BSNAME=foo, SIZES=[1 1 1], BSPARA=, BSARGS=, X0=0}
      mask prompts: BSNAME "Blockscript Name:"; BSPARA "Parameter Names:"; BSARGS "Blockscript Parameters:"; X0 "Initial Conditions:"
      mask help: BlockScript Programming Language.
      mask init: same as libsb2sl/USR/BlockScript
      mask Display: fprintf('Block\nScript')

== system libsb2sl/ALG/AlgExpression ==
  Constant : Subsystem  mask(ALG-Palette){SRC='y1=2.4;', P0=[]}
      mask prompts: SRC "Algebraic Equations:"; P0 "Initial Parameter Values:"
      mask help: Algebraic expressions.
      mask init:
      | if (exist('P0')==0),P0=[];end
      | [src,const]=sblibdrv('AlgebraicExp','constant',SRC,P0);
      mask Display: text(0.1,0.5,src,'HorizontalAlignment','left')
  General : S-Function  FunctionName=sbalgexp  Parameters=code,stat,data,info,P0,TS  EnableBusSupport=off  mask(ALG-Palette){SRC='y1=2.4;y2=t;', P0=[], TS=1}
      mask prompts: SRC "Algebraic Equations:"; P0 "Initial Parameter Values:"; TS "Sampling Period:"
      mask init:
      | if (exist('P0')==0),P0=[];end
      | [src,stat,code,data,info]=sblibdrv('AlgebraicExp','general',SRC,P0);
      mask Display: text(0.1,0.5,src,'HorizontalAlignment','left')
  General0 : libsb2sl/ALG/AlgExpression/General  SRC='y1=2.4;y2=t;'  P0=[]  TS=1
  Offset : Subsystem  mask(ALG-Palette){SRC='y1=2-u1;', P0=[]}
      mask prompts: SRC "Algebraic Equations:"; P0 "Initial Parameter Values:"
      mask help: Algebraic expressions.
      mask init:
      | if (exist('P0')==0),P0=[];end
      | [src,const,map,ni,sign]=sblibdrv('AlgebraicExp','offset',SRC,P0);
      mask Display: text(0.1,0.5,src,'HorizontalAlignment','left')
  PowerCU : Subsystem  mask(ALG-Palette){SRC='y1=2.4*u1;', P0=[]}
      mask prompts: SRC "Algebraic Equations:"; P0 "Initial Parameter Values:"
      mask help: Algebraic expressions.
      mask init:
      | if (exist('P0')==0),P0=[];end
      | [src,const,map,ni,sign]=sblibdrv('AlgebraicExp','powercu',SRC,P0);
      mask Display: text(0.1,0.5,src,'HorizontalAlignment','left')
  Product : Subsystem  mask(ALG-Palette){SRC='y1=u2*u1;', P0=[]}
      mask prompts: SRC "Algebraic Equations:"; P0 "Initial Parameter Values:"
      mask help: Algebraic expressions.
      mask init:
      | if (exist('P0')==0),P0=[];end
      | [src,sign,map,ni,oper]=sblibdrv('AlgebraicExp','product',SRC,P0);
      | set_param([gcb '/Product'],'Inputs',oper);
      mask Display: text(0.1,0.5,src,'HorizontalAlignment','left')
  Reciprocal : Subsystem  mask(ALG-Palette){SRC='y1=2.4/u1;', P0=[]}
      mask prompts: SRC "Algebraic Equations:"; P0 "Initial Parameter Values:"
      mask help: Algebraic expressions.
      mask init:
      | if (exist('P0')==0),P0=[];end
      | [src,const,map,ni]=sblibdrv('AlgebraicExp','reciprocal',SRC,P0);
      mask Display: text(0.1,0.5,src,'HorizontalAlignment','left')
  Scale : Subsystem  mask(ALG-Palette){SRC='y1=2.4*u1;', P0=[]}
      mask prompts: SRC "Algebraic Equations:"; P0 "Initial Parameter Values:"
      mask help: Algebraic expressions.
      mask init:
      | if (exist('P0')==0),P0=[];end
      | [src,gain,map,ni]=sblibdrv('AlgebraicExp','scale',SRC,P0);
      mask Display: text(0.1,0.5,src,'HorizontalAlignment','left')
  Summation : Subsystem  mask(ALG-Palette){SRC='y1=u2-u1;', P0=[]}
      mask prompts: SRC "Algebraic Equations:"; P0 "Initial Parameter Values:"
      mask help: Algebraic expressions.
      mask init:
      | if (exist('P0')==0),P0=[];end
      | [src,map,ni,sign]=sblibdrv('AlgebraicExp','summation',SRC,P0);
      mask Display: text(0.1,0.5,src,'HorizontalAlignment','left')

== system libsb2sl/ALG/CrossProd ==
  u1 : Inport  OutDataType=sfix(16)  OutScaling=2^0
  u2 : Inport  Port=2  OutDataType=sfix(16)  OutScaling=2^0
  Product : Product  OutDataType=sfix(16)  OutScaling=2^0  SaturateOnIntegerOverflow=on  RndMeth=Zero  InputSameDT=on  OutDataTypeStr=Inherit: Same as first input
  Product1 : Product  OutDataType=sfix(16)  OutScaling=2^0  SaturateOnIntegerOverflow=on  RndMeth=Zero  InputSameDT=on  OutDataTypeStr=Inherit: Same as first input
  Sum : Sum  Inputs=+-  OutDataType=sfix(16)  OutScaling=2^0  SaturateOnIntegerOverflow=on  InputSameDT=on  OutDataTypeStr=Inherit: Same as first input
  u1(231) : Selector  InputPortWidth=3  IndexOptions=Index vector (dialog)  Indices=[2 3 1]  OutputSizes=1
  u1(312) : Selector  InputPortWidth=3  IndexOptions=Index vector (dialog)  Indices=[3 1 2]  OutputSizes=1
  u2(231) : Selector  InputPortWidth=3  IndexOptions=Index vector (dialog)  Indices=[2 3 1]  OutputSizes=1
  u2(312) : Selector  InputPortWidth=3  IndexOptions=Index vector (dialog)  Indices=[3 1 2]  OutputSizes=1
  y : Outport  OutDataType=sfix(16)  OutScaling=2^0
  wires:
  u1(312)/1 -> Product1/1
  u2(231)/1 -> Product1/2
  Sum/1 -> y/1
  Product/1 -> Sum/1
  Product1/1 -> Sum/2
  u1/1 -> u1(231)/1, u1(312)/1
  u2/1 -> u2(312)/1, u2(231)/1
  u1(231)/1 -> Product/1
  u2(312)/1 -> Product/2

== system libsb2sl/ARC/BreakPoints ==
  u : Inport  OutDataType=sfix(16)  OutScaling=2^0
  Look-Up Table (n-D) : simulink3/Functions & Tables/Look-Up Table (n-D)  numDimsPopupSelect=1  bp1=in1BrkPoints  explicitNumDims=1  searchMode=Binary Search  cacheBpFlag=on  vectorInputFlag=on  tableData=outBrkPoints  interpMethod=Linear  extrapMethod=Linear  rangeErrorMode=None
  y : Outport  OutDataType=sfix(16)  OutScaling=2^0
  wires:
  Look-Up Table (n-D)/1 -> y/1
  u/1 -> Look-Up Table (n-D)/1

== system libsb2sl/ARC/InterpTable ==
  u : Inport  OutDataType=sfix(16)  OutScaling=2^0
  sblininterp : S-Function  FunctionName=sblintable  Parameters=numInp,in1BrkPoints,in2BrkPoints,outBrkPoints  EnableBusSupport=off
  y : Outport  OutDataType=sfix(16)  OutScaling=2^0
  wires:
  sblininterp/1 -> y/1
  u/1 -> sblininterp/1

== system libsb2sl/DYN/CBacklash ==
  u : Inport  OutDataType=sfix(16)  OutScaling=2^0
  Dead Zone : DeadZone  LowerValue=lb  UpperValue=ub  SaturateOnIntegerOverflow=on
  Gain1 : Gain  Gain=N  ParameterDataType=sfix(16)  ParameterScaling=2^0  OutDataType=sfix(16)  OutScaling=2^0  SaturateOnIntegerOverflow=on  OutDataTypeStr=Inherit: Same as input  ParamDataTypeStr=Inherit: Same as input
  Integrator : Integrator  InitialCondition=X0
  Sum2 : Sum  Inputs=+-  OutDataType=sfix(16)  OutScaling=2^0  SaturateOnIntegerOverflow=on  InputSameDT=on  OutDataTypeStr=Inherit: Same as first input
  wc : Gain  Gain=Wc  ParameterDataType=sfix(16)  ParameterScaling=2^0  OutDataType=sfix(16)  OutScaling=2^0  SaturateOnIntegerOverflow=on  OutDataTypeStr=Inherit: Same as input  ParamDataTypeStr=Inherit: Same as input
  y : Outport  OutDataType=sfix(16)  OutScaling=2^0
  wires:
  Dead Zone/1 -> wc/1
  wc/1 -> Integrator/1
  Sum2/1 -> Dead Zone/1
  Integrator/1 -> Gain1/1, Sum2/2
  u/1 -> Sum2/1
  Gain1/1 -> y/1

== system libsb2sl/DYN/CGainDampsFreqs ==
  u : Inport  OutDataType=sfix(16)  OutScaling=2^0
  State Space : StateSpace  A=A  B=B  C=C  D=D  X0=X0
  y : Outport  OutDataType=sfix(16)  OutScaling=2^0
  wires:
  State Space/1 -> y/1
  u/1 -> State Space/1

== system libsb2sl/DYN/CGainZerosPoles ==
  u : Inport  OutDataType=sfix(16)  OutScaling=2^0
  State Space : StateSpace  A=A  B=B  C=C  D=D  X0=X0
  y : Outport  OutDataType=sfix(16)  OutScaling=2^0
  wires:
  State Space/1 -> y/1
  u/1 -> State Space/1

== system libsb2sl/DYN/CIntegrator ==
  1stOrder : Subsystem  mask(DYN-Palette){K=1, X0=0}
      mask prompts: K "Output Gains:"; X0 "Initial Conditions:"
      mask help: Nth order integration of an input.
      mask init:
      | [x,y]=sblibico('1stOrderInteg','cont');
      mask Display: plot(0,0,1,1,x,y)
  NthOrder : Subsystem  mask(DYN-Palette){N=1, K=1, X0=0}
      mask prompts: N "Order of Integration:"; K "Output Gains:"; X0 "Initial Conditions:"
      mask help: Nth order integration of an input.
      mask init:
      | no=length(K);
      | stateMap=sblibdrv('Integrator',N,no,0);
      | [x,y]=sblibico('nthOrderInteg','cont');
      mask Display: plot(0,0,1,1,x,y)
  NthOrder1 : Subsystem  mask(DYN-Palette){N=1, X0=0}
      mask prompts: N "Order of Integration:"; X0 "Initial Conditions:"
      mask help: Nth order integration of an input.
      mask init:
      | no=length(X0)/N;
      | stateMap=sblibdrv('Integrator',N,no,0);
      | [x,y]=sblibico('nthOrder1Integ','cont');
      mask Display: plot(0,0,1,1,x,y)

== system libsb2sl/DYN/CLimInt ==
  u : Inport  OutDataType=sfix(16)  OutScaling=2^0
  Gain : Gain  Gain=K  ParameterDataType=sfix(16)  ParameterScaling=2^0  OutDataType=sfix(16)  OutScaling=2^0  SaturateOnIntegerOverflow=on  OutDataTypeStr=Inherit: Same as input  ParamDataTypeStr=Inherit: Same as input
  Integrator : Integrator  InitialCondition=X0  LimitOutput=on  UpperSaturationLimit=UB  LowerSaturationLimit=LB
  y : Outport  OutDataType=sfix(16)  OutScaling=2^0
  wires:
  Integrator/1 -> Gain/1
  Gain/1 -> y/1
  u/1 -> Integrator/1

== system libsb2sl/DYN/CNumDenCoeffs ==
  u : Inport  OutDataType=sfix(16)  OutScaling=2^0
  State Space : StateSpace  A=Ac  B=Bc  C=Cc  D=Dc  X0=X0
  y : Outport  OutDataType=sfix(16)  OutScaling=2^0
  wires:
  u/1 -> State Space/1
  State Space/1 -> y/1

== system libsb2sl/DYN/CPIDControlLaw ==
  e : Inport  OutDataType=sfix(16)  OutScaling=2^0
  D Term : Subsystem  TreatAsAtomicUnit=on
  I Term : Subsystem  TreatAsAtomicUnit=on
  Proportional : Gain  Gain=P  ParameterDataType=sfix(16)  ParameterScaling=2^0  OutDataType=sfix(16)  OutScaling=2^0  SaturateOnIntegerOverflow=on  OutDataTypeStr=Inherit: Same as input  ParamDataTypeStr=Inherit: Same as input
  Sum : Sum  Inputs=+++  OutDataType=sfix(16)  OutScaling=2^0  SaturateOnIntegerOverflow=on  InputSameDT=on  OutDataTypeStr=Inherit: Same as first input
  ed : Constant  Value=D ~= 0  OutDataType=sfix(16)  OutScaling=2^0
  ei : Constant  Value=I ~= 0  OutDataType=sfix(16)  OutScaling=2^0
  u : Outport  OutDataType=sfix(16)  OutScaling=2^0
  wires:
  e/1 -> Proportional/1, D Term/1(e), I Term/1(e)
  Proportional/1 -> Sum/1
  Sum/1 -> u/1
  I Term/1(u_i) -> Sum/2
  D Term/1(u_d) -> Sum/3
  ed/1 -> D Term/Enable
  ei/1 -> I Term/Enable

== system libsb2sl/DYN/CResetIntegrator ==
  1stOrder : Subsystem  mask(DYN-Palette){RMODE=Single edge, K=1, X0=0}
      mask prompts: RMODE "External Reset:"; K "Output Gains:"; X0 "Initial Conditions:"
      mask help: Nth order integration of an input with resettable states.
      mask init:
      | operator={'rising','either'};
      | set_param([gcb '/Integrator'],'ExternalReset',operator{RMODE});
      | [x,y]=sblibico('1stOrderReset','cont');
      mask StyleString: popup(Single edge|Double edge),edit,edit
      mask Display: plot(0,0,1,1,x,y)
  1stOrder1 : Subsystem  mask(DYN-Palette){RMODE=Single edge, X0=0}
      mask prompts: RMODE "External Reset:"; X0 "Initial Conditions:"
      mask help: Nth order integration of an input with resettable states.
      mask init:
      | operator={'rising','either'};
      | set_param([gcb '/Integrator'],'ExternalReset',operator{RMODE});
      | [x,y]=sblibico('1stOrder1Reset','cont');
      mask StyleString: popup(Single edge|Double edge),edit
      mask Display: plot(0,0,1,1,x,y)
  NthOrder : Subsystem  mask(DYN-Palette){N=1, RMODE=Single edge, NR=1, K=1, X0=0}
      mask prompts: N "Order of Integration:"; RMODE "External Reset:"; NR "Highest Order of  Resettable State:"; K "Output Gains:"; X0 "Initial Conditions:"
      mask help: Nth order integration of an input with resettable states.
      mask init:
      | no=length(K);
      | [stateMap,resetMap]=sblibdrv('Integrator',N,no,NR);
      | operator={'rising','either'};
      | set_param([gcb '/Integrator'],'ExternalReset',operator{RMODE});
      | [x,y]=sblibico('nthOrderReset','cont');
      mask StyleString: edit,popup(Single edge|Double edge),edit,edit,edit
      mask Display: plot(0,0,1,1,x,y)
  NthOrder1 : Subsystem  mask(DYN-Palette){N=1, RMODE=Single edge, NR=1, X0=0}
      mask prompts: N "Order of Integration:"; RMODE "External Reset:"; NR "Highest Order of  Resettable State:"; X0 "Initial Conditions:"
      mask help: Nth order integration of an input with resettable states.
      mask init:
      | no=length(X0)/N;
      | [stateMap,resetMap]=sblibdrv('Integrator',N,no,NR);
      | operator={'rising','either'};
      | set_param([gcb '/Integrator'],'ExternalReset',operator{RMODE});
      | [x,y]=sblibico('nthOrder1Reset','cont');
      mask StyleString: edit,popup(Single edge|Double edge),edit,edit
      mask Display: plot(0,0,1,1,x,y)

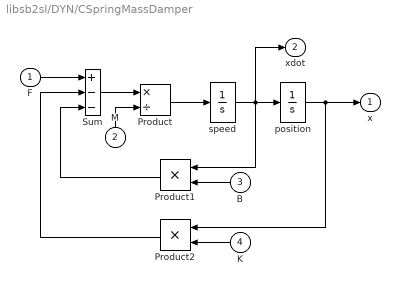
== system libsb2sl/DYN/CSpringMassDamper ==
  F : Inport  OutDataType=sfix(16)  OutScaling=2^0
  M : Inport  Port=2  OutDataType=sfix(16)  OutScaling=2^0
  B : Inport  Port=3  OutDataType=sfix(16)  OutScaling=2^0
  K : Inport  Port=4  OutDataType=sfix(16)  OutScaling=2^0
  Product : Product  Inputs=*/  OutDataType=sfix(16)  OutScaling=2^0  SaturateOnIntegerOverflow=on  RndMeth=Zero  InputSameDT=on  OutDataTypeStr=Inherit: Same as first input
  Product1 : Product  OutDataType=sfix(16)  OutScaling=2^0  SaturateOnIntegerOverflow=on  RndMeth=Zero  InputSameDT=on  OutDataTypeStr=Inherit: Same as first input
  Product2 : Product  OutDataType=sfix(16)  OutScaling=2^0  SaturateOnIntegerOverflow=on  RndMeth=Zero  InputSameDT=on  OutDataTypeStr=Inherit: Same as first input
  Sum : Sum  Inputs=+--  OutDataType=sfix(16)  OutScaling=2^0  SaturateOnIntegerOverflow=on  InputSameDT=on  OutDataTypeStr=Inherit: Same as first input
  position : Integrator  InitialCondition=X0(1)
  speed : Integrator  InitialCondition=X0(2)
  x : Outport  OutDataType=sfix(16)  OutScaling=2^0
  xdot : Outport  Port=2  OutDataType=sfix(16)  OutScaling=2^0
  wires:
  K/1 -> Product2/2
  B/1 -> Product1/2
  M/1 -> Product/2
  position/1 -> Product2/1, x/1
  F/1 -> Sum/1
  Product2/1 -> Sum/2
  Product1/1 -> Sum/3
  speed/1 -> xdot/1, Product1/1, position/1
  Product/1 -> speed/1
  Sum/1 -> Product/1

== system libsb2sl/DYN/CStateSpace ==
  u : Inport  OutDataType=sfix(16)  OutScaling=2^0
  StateSpace : StateSpace  A=A  B=B  C=C  D=D  X0=X0
  y : Outport  OutDataType=sfix(16)  OutScaling=2^0
  wires:
  u/1 -> StateSpace/1
  StateSpace/1 -> y/1

== system libsb2sl/DYN/DBacklash ==
  u : Inport  SampleTime=TS  OutDataType=sfix(16)  OutScaling=2^0
  Dead Zone : DeadZone  LowerValue=lb  UpperValue=ub  SaturateOnIntegerOverflow=on
  Gain1 : Gain  Gain=N  ParameterDataType=sfix(16)  ParameterScaling=2^0  OutDataType=sfix(16)  OutScaling=2^0  SaturateOnIntegerOverflow=on  OutDataTypeStr=Inherit: Same as input  ParamDataTypeStr=Inherit: Same as input
  Sum2 : Sum  Inputs=|+-  OutDataType=sfix(16)  OutScaling=2^0  SaturateOnIntegerOverflow=on  InputSameDT=on  OutDataTypeStr=Inherit: Same as first input
  Sum3 : Sum  Inputs=|++  OutDataType=sfix(16)  OutScaling=2^0  SaturateOnIntegerOverflow=on  InputSameDT=on  OutDataTypeStr=Inherit: Same as first input
  Unit Delay : UnitDelay  X0=X0  SampleTime=TS
  y : Outport  OutDataType=sfix(16)  OutScaling=2^0
  wires:
  Unit Delay/1 -> Sum3/2, Sum2/2
  u/1 -> Sum2/1
  Sum2/1 -> Dead Zone/1
  Dead Zone/1 -> Sum3/1
  Gain1/1 -> y/1
  Sum3/1 -> Gain1/1, Unit Delay/1

== system libsb2sl/DYN/DGainDampsFreqs ==
  u : Inport  SampleTime=TS  OutDataType=sfix(16)  OutScaling=2^0
  Discrete State Space : DiscreteStateSpace  A=A  B=B  C=C  D=D  X0=X0  SampleTime=TS
  y : Outport  OutDataType=sfix(16)  OutScaling=2^0
  wires:
  u/1 -> Discrete State Space/1
  Discrete State Space/1 -> y/1

== system libsb2sl/DYN/DGainZerosPoles ==
  u : Inport  SampleTime=TS  OutDataType=sfix(16)  OutScaling=2^0
  Discrete State Space : DiscreteStateSpace  A=A  B=B  C=C  D=D  X0=X0  SampleTime=TS
  y : Outport  OutDataType=sfix(16)  OutScaling=2^0
  wires:
  u/1 -> Discrete State Space/1
  Discrete State Space/1 -> y/1

== system libsb2sl/DYN/DIntegrator ==
  1stOrder : Subsystem  mask(DYN-Palette){IMODE=Forward Euler, K=1, X0=0, TS=0.1}
      mask prompts: IMODE "Integrator Method:"; K "Output Gains:"; X0 "Initial Conditions:"; TS "Sampling Time:"
      mask help: Nth order integration of an input.
      mask init:
      | method={'ForwardEuler';'BackwardEuler';'Trapezoidal'};
      | set_param([gcb '/Integrator'],'IntegratorMethod',method{IMODE});
      | [x,y]=sblibico('1stOrderInteg','disc');
      mask StyleString: popup(Forward Euler|Backward Euler|Trapezoidal),edit,edit,edit
      mask Display: plot(0,0,1,1,x,y)
  NthOrder : Subsystem  mask(DYN-Palette){IMODE=Forward Euler, N=1, K=1, X0=0, TS=0.1}
      mask prompts: IMODE "Integrator Method:"; N "Order of Integration:"; K "Output Gains:"; X0 "Initial Conditions:"; TS "Sampling Time:"
      mask help: Nth order integration of an input.
      mask init:
      | no=length(K);
      | stateMap=sblibdrv('Integrator',N,no,0);
      | method={'ForwardEuler';'BackwardEuler';'Trapezoidal'};
      | set_param([gcb '/Integrator'],'IntegratorMethod',method{IMODE});
      | [x,y]=sblibico('nthOrderInteg','disc');
      mask StyleString: popup(Forward Euler|Backward Euler|Trapezoidal),edit,edit,edit,edit
      mask Display: plot(0,0,1,1,x,y)
  NthOrder1 : Subsystem  mask(DYN-Palette){IMODE=Forward Euler, N=1, X0=0, TS=0.1}
      mask prompts: IMODE "Integrator Method:"; N "Order of Integration:"; X0 "Initial Conditions:"; TS "Sampling Time:"
      mask help: Nth order integration of an input.
      mask init:
      | no=length(X0)/N;
      | stateMap=sblibdrv('Integrator',N,no,0);
      | method={'ForwardEuler';'BackwardEuler';'Trapezoidal'};
      | set_param([gcb '/Integrator'],'IntegratorMethod',method{IMODE});
      | [x,y]=sblibico('nthOrder1Integ','disc');
      mask StyleString: popup(Forward Euler|Backward Euler|Trapezoidal),edit,edit,edit
      mask Display: plot(0,0,1,1,x,y)

== system libsb2sl/DYN/DLimInt ==
  u : Inport  SampleTime=TS  OutDataType=sfix(16)  OutScaling=2^0
  Gain : Gain  Gain=K  ParameterDataType=sfix(16)  ParameterScaling=2^0  OutDataType=sfix(16)  OutScaling=2^0  SaturateOnIntegerOverflow=on  OutDataTypeStr=Inherit: Same as input  ParamDataTypeStr=Inherit: Same as input
  Integrator : DiscreteIntegrator  InitialCondition=X0  SampleTime=TS  OutDataType=sfix(16)  OutScaling=2^0  LimitOutput=on  UpperSaturationLimit=UB  LowerSaturationLimit=LB  ICPrevOutput=DiscIntNeverNeededParam  ICPrevScaledInput=DiscIntNeverNeededParam
  y : Outport  OutDataType=sfix(16)  OutScaling=2^0
  wires:
  Gain/1 -> y/1
  u/1 -> Integrator/1
  Integrator/1 -> Gain/1

== system libsb2sl/DYN/DNumDenCoeffs ==
  u : Inport  SampleTime=TS  OutDataType=sfix(16)  OutScaling=2^0
  Discrete State Space : DiscreteStateSpace  A=Ad  B=Bd  C=Cd  D=Dd  X0=X0  SampleTime=TS
  y : Outport  OutDataType=sfix(16)  OutScaling=2^0
  wires:
  Discrete State Space/1 -> y/1
  u/1 -> Discrete State Space/1

== system libsb2sl/DYN/DPIDControlLaw ==
  e : Inport  SampleTime=TS  OutDataType=sfix(16)  OutScaling=2^0
  D Term : Subsystem  TreatAsAtomicUnit=on
  I Term : Subsystem  TreatAsAtomicUnit=on
  Proportional : Gain  Gain=P  ParameterDataType=sfix(16)  ParameterScaling=2^0  OutDataType=sfix(16)  OutScaling=2^0  SaturateOnIntegerOverflow=on  OutDataTypeStr=Inherit: Same as input  ParamDataTypeStr=Inherit: Same as input
  Sum : Sum  Inputs=+++  OutDataType=sfix(16)  OutScaling=2^0  SaturateOnIntegerOverflow=on  InputSameDT=on  OutDataTypeStr=Inherit: Same as first input
  ed : Constant  Value=D ~= 0  OutDataType=sfix(16)  OutScaling=2^0
  ei : Constant  Value=I ~= 0  OutDataType=sfix(16)  OutScaling=2^0
  u : Outport  OutDataType=sfix(16)  OutScaling=2^0
  wires:
  e/1 -> Proportional/1, D Term/1(e), I Term/1(e)
  Sum/1 -> u/1
  D Term/1(u_d) -> Sum/3
  I Term/1(u_i) -> Sum/2
  Proportional/1 -> Sum/1
  ed/1 -> D Term/Enable
  ei/1 -> I Term/Enable
